simulink subsystem "DirectDriveCycleRefSub"  (R2020b)
settings: Solver=VariableStepAuto  StartTime=0.0  StopTime=10.0  RelTol=1e-3
undefined symbols (not defined in the file): batteryHV, bevMotorSpdRef, motorDrive, vehicle
libraries: autolibshared x1
settings Model: Creator=isaacito  LastModifiedBy=isaacito

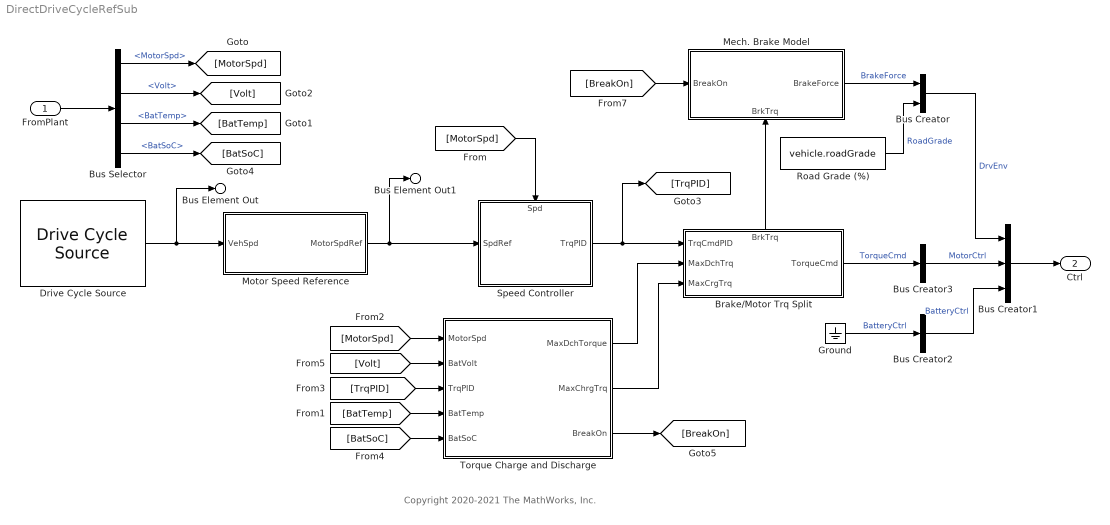
== system DirectDriveCycleRefSub ==
  note: Copyright 2020-2021 The MathWorks, Inc.
  FromPlant : Inport
  Brake/Motor Trq Split : Subsystem
      settings: PortSchema="{\"entries\":[{\"content\":{\"sides\":[{\"content\":{\"connectorIds\":[\"In1\",\"In2\",\"In3\"]},\"type\":\"ConnectorPlacement.EquallySpacedRectSide\",\"uuid\":\"c6883188-188e-4cbf-9dc5-1a26bf01b714\"},{\"content\":{\"connectorIds\":[\"Out1\"],\"side\":\"RIGHT\"},\"type\":\"ConnectorPlacement.EquallySpacedRectSide\",\"uuid\":\"b7c90991-838b-485d-9a4c-3fbacac28b54\"},{\"content\":{\"connectorIds\":[\"Out2\"],\"side\":\"TOP\"},\"type\":\"ConnectorPlacement.EquallySpacedRectSide\",\"uuid\":\"50e43671-3241-4bf5-a3b9-e23b27b7214a\"},{\"content\":{\"connectorIds\":[],\"side\":\"HIDDEN\"},\"type\":\"ConnectorPlacement.EquallySpacedRectSide\",\"uuid\":\"7c25a71e-e9cc-425c-8a3d-1b4aa412427f\"}]},\"type\":\"ConnectorPlacement.EquallySpacedConnector\",\"uuid\":\"d51dcaef-c892-4ef2-982d-c6c52760ceaa\"}],\"packageUris\":[\"http://schema.mathworks.com/mf0/Connector/R2020b\"],\"version\":\"1.0\"}"
  Bus Creator : BusCreator  Inputs=2
  Bus Creator1 : BusCreator  Inputs=3
  Bus Creator2 : BusCreator  Inputs=1
  Bus Creator3 : BusCreator  Inputs=1
  Bus Selector : BusSelector  OutputSignals=Motor.MotorSpd,Battery.Volt,Battery.BatTemp,Battery.BatSoC
  Drive Cycle Source : autolibshared/Drive Cycle Source  cycleVar=FTP75  fileVar=cycleFTP75.mat  tfinal="2474  seconds"  cycleRepeat=off  outAccPort=off  outGearPort=off  gearList=No gear data  t_wot1=5  xdot_woto=0  xdot_wot1=30  t_wot2=20  xdot_wot2=0  t_wotend=30  srcUnit=m/s  outUnit=km/h  srcAccUnit=m/s/s  outAccUnit=m/s^2  dt=0  aMode=1  faultOption=off  velBnd=2  velBndUnit=mph  inUnit=m/s  timeBnd=1  failOption=off  stopSim=off  maxFaultCnt=10  maxFaultTime=2  maxTotFaultTime=15  traceOption=off  dtTrace=1  traceWindow=10  lastDCname=FTP75  lastOutUnit=mph  lastDT=0  lastTB=1  lastSB=2  forceCalcBound=off
      settings: SourceProductBaseCode=PW,MT,VE,VP
  Ground : Ground
  Mech. Brake Model : Subsystem
      settings: PortSchema="{\"entries\":[{\"content\":{\"sides\":[{\"content\":{\"connectorIds\":[\"In1\"]},\"type\":\"ConnectorPlacement.EquallySpacedRectSide\",\"uuid\":\"3fcf8e06-a346-49b8-a4a8-b41cf2b27013\"},{\"content\":{\"connectorIds\":[\"Out1\"],\"side\":\"RIGHT\"},\"type\":\"ConnectorPlacement.EquallySpacedRectSide\",\"uuid\":\"8698242e-d004-4fda-889c-69f0784e7402\"},{\"content\":{\"connectorIds\":[],\"side\":\"TOP\"},\"type\":\"ConnectorPlacement.EquallySpacedRectSide\",\"uuid\":\"7829013b-7288-42bb-bccf-7e6edbe20d12\"},{\"content\":{\"connectorIds\":[\"In2\"],\"side\":\"BOTTOM\"},\"type\":\"ConnectorPlacement.EquallySpacedRectSide\",\"uuid\":\"357a4631-0a09-454f-b0f2-2b693ca62a9f\"},{\"content\":{\"connectorIds\":[],\"side\":\"HIDDEN\"},\"type\":\"ConnectorPlacement.EquallySpacedRectSide\",\"uuid\":\"b5eacf60-b578-4936-bef0-d59a279d5824\"}]},\"type\":\"ConnectorPlacement.EquallySpacedConnector\",\"uuid\":\"d2ebf12e-a3e7-4a55-b8c6-fa4e5ed13b89\"}],\"packageUris\":[\"http://schema.mathworks.com/mf0/Connector/R2020b\"],\"version\":\"1.0\"}"
  Motor Speed Reference : Subsystem
  Road Grade (%) : Constant  Value=vehicle.roadGrade
  Speed Controller : Subsystem
      settings: PortSchema="{\"entries\":[{\"content\":{\"sides\":[{\"content\":{\"connectorIds\":[\"Out1\"]},\"type\":\"ConnectorPlacement.EquallySpacedRectSide\",\"uuid\":\"12b9f2c9-2b28-451b-ad36-7fe4150db485\"},{\"content\":{\"connectorIds\":[\"In2\"],\"side\":\"RIGHT\"},\"type\":\"ConnectorPlacement.EquallySpacedRectSide\",\"uuid\":\"c0fdf9a4-483a-4ddc-b663-6299fcc79327\"},{\"content\":{\"connectorIds\":[\"In1\"],\"side\":\"TOP\"},\"type\":\"ConnectorPlacement.EquallySpacedRectSide\",\"uuid\":\"3f20082e-8487-45e3-9fd7-d6d75741df4d\"}]},\"type\":\"ConnectorPlacement.EquallySpacedConnector\",\"uuid\":\"9361cdd3-74d8-46ee-ae7f-e2dde5d31ed1\"}],\"packageUris\":[\"http://schema.mathworks.com/mf0/Connector/19700101\"],\"version\":\"1.0\"}"
  Torque Charge and Discharge : Subsystem
  Bus Element Out : Outport  PortName=Info  Element=VehSpdRef
      settings: AttributesFormatString=%<Unit>
  Bus Element Out1 : Outport  PortName=Info  Element=MotorSpdRef
      settings: AttributesFormatString=%<Unit>
  Ctrl : Outport  Port=2
  wires:
  Drive Cycle Source/1 -> Bus Element Out/1, Motor Speed Reference/1(VehSpd)
  Motor Speed Reference/1(MotorSpdRef) -> Bus Element Out1/1, Speed Controller/2(SpdRef)
  Road Grade (%)/1 -> Bus Creator/2  "RoadGrade"
  [MotorSpd] -> Speed Controller/1(Spd)
  FromPlant/1 -> Bus Selector/1
  Bus Selector/1 -> [MotorSpd]  "<MotorSpd>"
  Ground/1 -> Bus Creator2/1  "BatteryCtrl"
  Bus Creator/1 -> Bus Creator1/1  "DrvEnv"
  Bus Creator3/1 -> Bus Creator1/2  "MotorCtrl"
  Bus Creator2/1 -> Bus Creator1/3  "BatteryCtrl"
  Bus Creator1/1 -> Ctrl/1
  Bus Selector/2 -> [Volt]  "<Volt>"
  Speed Controller/1(TrqPID) -> Brake/Motor Trq Split/1(TrqCmdPID), [TrqPID]
  Torque Charge and Discharge/3(BreakOn) -> [BreakOn]
  [MotorSpd] -> Torque Charge and Discharge/1(MotorSpd)
  [Volt] -> Torque Charge and Discharge/2(BatVolt)
  [TrqPID] -> Torque Charge and Discharge/3(TrqPID)
  Mech. Brake Model/1(BrakeForce) -> Bus Creator/1  "BrakeForce"
  [BreakOn] -> Mech. Brake Model/1(BreakOn)
  Torque Charge and Discharge/1(MaxDchTorque) -> Brake/Motor Trq Split/2(MaxDchTrq)
  Torque Charge and Discharge/2(MaxChrgTrq) -> Brake/Motor Trq Split/3(MaxCrgTrq)
  Brake/Motor Trq Split/2(BrkTrq) -> Mech. Brake Model/2(BrkTrq)
  Brake/Motor Trq Split/1(TorqueCmd) -> Bus Creator3/1  "TorqueCmd"
  Bus Selector/3 -> [BatTemp]  "<BatTemp>"
  Bus Selector/4 -> [BatSoC]  "<BatSoC>"
  [BatTemp] -> Torque Charge and Discharge/4(BatTemp)
  [BatSoC] -> Torque Charge and Discharge/5(BatSoC)

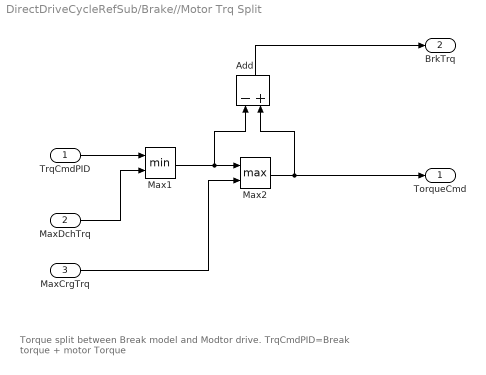
== system DirectDriveCycleRefSub/Brake//Motor Trq Split ==
  note: Torque split between Break model and Modtor drive.
      | TrqCmdPID=Break torque + motor Torque
  TrqCmdPID : Inport
  MaxDchTrq : Inport  Port=2
  MaxCrgTrq : Inport  Port=3
  Add : Sum  Inputs=-+
  Max1 : MinMax  Inputs=2  ZeroCross=off
  Max2 : MinMax  Function=max  Inputs=2  ZeroCross=off
  TorqueCmd : Outport
  BrkTrq : Outport  Port=2
  wires:
  MaxDchTrq/1 -> Max1/2
  Max2/1 -> Add/2, TorqueCmd/1
  Add/1 -> BrkTrq/1
  Max1/1 -> Add/1, Max2/1
  TrqCmdPID/1 -> Max1/1
  MaxCrgTrq/1 -> Max2/2

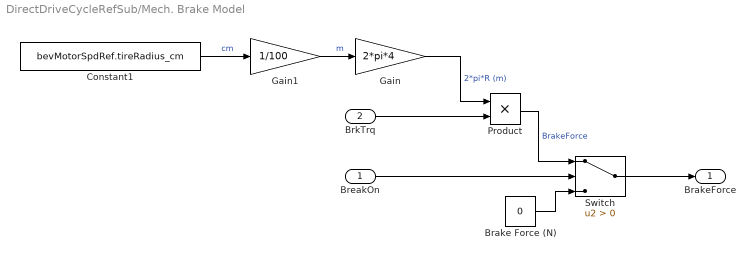
== system DirectDriveCycleRefSub/Mech. Brake Model ==
  BreakOn : Inport
  BrkTrq : Inport  Port=2
  Brake Force (N) : Constant  Value=0
  Constant1 : Constant  Value=bevMotorSpdRef.tireRadius_cm
  Gain : Gain  Gain=2*pi*4
  Gain1 : Gain  Gain=1/100
  Product : Product
  Switch : Switch  Criteria=u2 > Threshold  ZeroCross=off
  BrakeForce : Outport
  wires:
  Switch/1 -> BrakeForce/1
  Gain1/1 -> Gain/1  "m"
  Brake Force (N)/1 -> Switch/3
  BreakOn/1 -> Switch/2
  BrkTrq/1 -> Product/2
  Gain/1 -> Product/1  "2*pi*R (m)"
  Constant1/1 -> Gain1/1  "cm"
  Product/1 -> Switch/1  "BrakeForce"

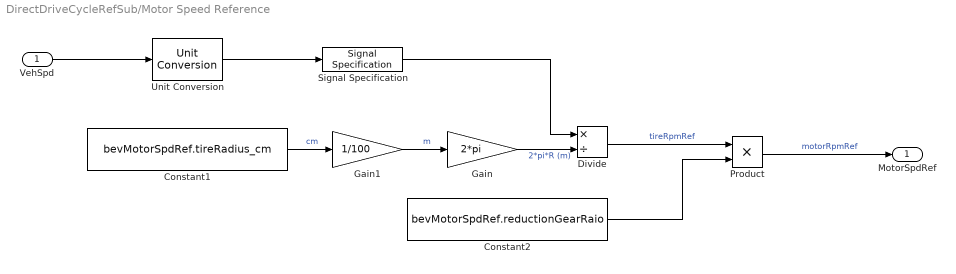
== system DirectDriveCycleRefSub/Motor Speed Reference ==
  VehSpd : Inport  Unit=km/hr
  Constant1 : Constant  Value=bevMotorSpdRef.tireRadius_cm
  Constant2 : Constant  Value=bevMotorSpdRef.reductionGearRaio
  Divide : Product  Inputs=*/
  Gain : Gain  Gain=2*pi
  Gain1 : Gain  Gain=1/100
  Product : Product
  Signal Specification : SignalSpecification  Unit=m/min
  Unit Conversion : UnitConversion
  MotorSpdRef : Outport  Unit=rpm  VectorParamsAs1DForOutWhenUnconnected=off
  wires:
  Gain1/1 -> Gain/1  "m"
  Product/1 -> MotorSpdRef/1  "motorRpmRef"
  Constant2/1 -> Product/2
  Divide/1 -> Product/1  "tireRpmRef"
  Gain/1 -> Divide/2  "2*pi*R (m)"
  Constant1/1 -> Gain1/1  "cm"
  Signal Specification/1 -> Divide/1
  Unit Conversion/1 -> Signal Specification/1
  VehSpd/1 -> Unit Conversion/1

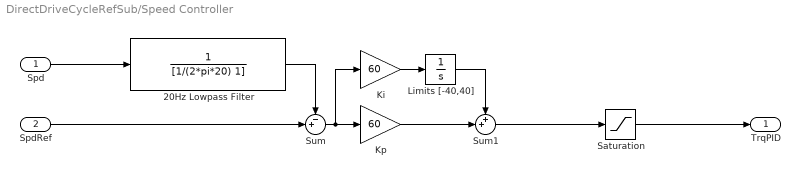
== system DirectDriveCycleRefSub/Speed Controller ==
  Spd : Inport  Unit=rpm
      settings: AttributesFormatString=%<Unit>
  SpdRef : Inport  Port=2  Unit=rpm
      settings: AttributesFormatString=%<Unit>
  20Hz Lowpass Filter : TransferFcn  Denominator=[1/(2*pi*20) 1]
  Ki : Gain  Gain=60
  Kp : Gain  Gain=60
  Limits [-40,40] : Integrator  LimitOutput=on  UpperSaturationLimit=40  LowerSaturationLimit=-40
  Saturation : Saturate  UpperLimit=motorDrive.simplePmsmDrv_trqMax_Nm  LowerLimit=-motorDrive.simplePmsmDrv_trqMax_Nm
      settings: AttributesFormatString=|
      | %<UpperLimit>
      | %<LowerLimit>
  Sum : Sum  Inputs=-+|
  Sum1 : Sum  Inputs=++|
  TrqPID : Outport  Unit=N*m  VectorParamsAs1DForOutWhenUnconnected=off
      settings: AttributesFormatString=%<Unit>
  wires:
  SpdRef/1 -> Sum/2
  Spd/1 -> 20Hz Lowpass Filter/1
  Sum1/1 -> Saturation/1
  Sum/1 -> Ki/1, Kp/1
  Ki/1 -> Limits [-40,40]/1
  Kp/1 -> Sum1/2
  Limits [-40,40]/1 -> Sum1/1
  20Hz Lowpass Filter/1 -> Sum/1
  Saturation/1 -> TrqPID/1

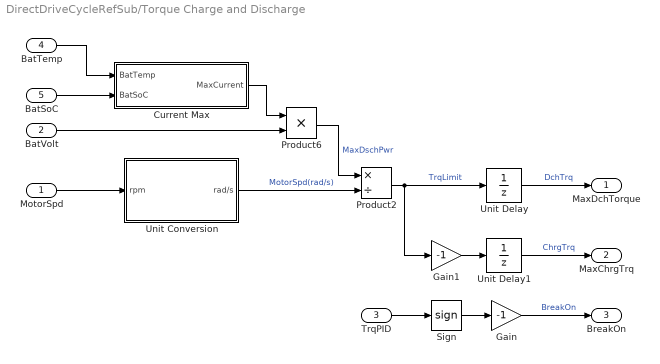
== system DirectDriveCycleRefSub/Torque Charge and Discharge ==
  MotorSpd : Inport
  BatVolt : Inport  Port=2
  TrqPID : Inport  Port=3
  BatTemp : Inport  Port=4
  BatSoC : Inport  Port=5
  Current Max : Subsystem
  Gain : Gain  Gain=-1
  Gain1 : Gain  Gain=-1
  Product2 : Product  Inputs=*/
  Product6 : Product
  Sign : Signum  ZeroCross=off
  Unit Conversion : Subsystem
  Unit Delay : UnitDelay  InitialCondition=eps  SampleTime=-1  HasFrameUpgradeWarning=on
  Unit Delay1 : UnitDelay  InitialCondition=eps  SampleTime=-1  HasFrameUpgradeWarning=on
  MaxDchTorque : Outport
  MaxChrgTrq : Outport  Port=2
  BreakOn : Outport  Port=3
  wires:
  Gain1/1 -> Unit Delay1/1
  Current Max/1(MaxCurrent) -> Product6/1
  BatSoC/1 -> Current Max/2(BatSoC)
  BatTemp/1 -> Current Max/1(BatTemp)
  MotorSpd/1 -> Unit Conversion/1(rpm)
  Unit Conversion/1(rad/s) -> Product2/2  "MotorSpd(rad/s)"
  Product6/1 -> Product2/1  "MaxDschPwr"
  Product2/1 -> Unit Delay/1, Gain1/1  "TrqLimit"
  BatVolt/1 -> Product6/2
  Sign/1 -> Gain/1
  TrqPID/1 -> Sign/1
  Unit Delay1/1 -> MaxChrgTrq/1  "ChrgTrq"
  Gain/1 -> BreakOn/1  "BreakOn"
  Unit Delay/1 -> MaxDchTorque/1  "DchTrq"

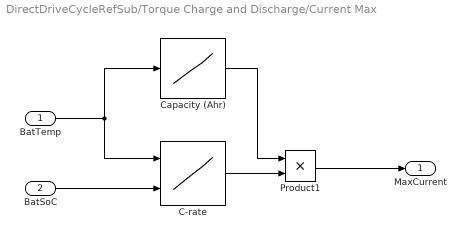
== system DirectDriveCycleRefSub/Torque Charge and Discharge/Current Max ==
  BatTemp : Inport
  BatSoC : Inport  Port=2
  C-rate : Lookup_n-D  BreakpointsForDimension1=batteryHV.batteryTemp_LUT  BreakpointsForDimension2=batteryHV.batterySOC_LUT  Table=batteryHV.cRate'  ExtrapMethod=Clip  UseLastTableValue=on  InternalRulePriority=Speed  RndMeth=Simplest  InputSameDT=on
      settings: InputPortMap=u0,u1
  Capacity (Ahr) : Lookup_n-D  NumberOfTableDimensions=1  BreakpointsForDimension1=batteryHV.batteryTemp_LUT  Table=batteryHV.batteryCapacity_LUT.*batteryHV.batteryNp  ExtrapMethod=Clip  UseLastTableValue=on  InternalRulePriority=Speed  RndMeth=Simplest  InputSameDT=on
  Product1 : Product
  MaxCurrent : Outport
  wires:
  Capacity (Ahr)/1 -> Product1/1
  BatSoC/1 -> C-rate/2
  BatTemp/1 -> Capacity (Ahr)/1, C-rate/1
  Product1/1 -> MaxCurrent/1
  C-rate/1 -> Product1/2

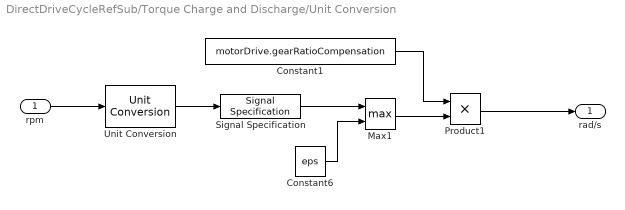
== system DirectDriveCycleRefSub/Torque Charge and Discharge/Unit Conversion ==
  rpm : Inport
  Constant1 : Constant  Value=motorDrive.gearRatioCompensation
  Constant6 : Constant  Value=eps
  Max1 : MinMax  Function=max  Inputs=2  ZeroCross=off
  Product1 : Product
  Signal Specification : SignalSpecification  OutMin=[0]  Unit=rad/sec
  Unit Conversion : UnitConversion
  rad/s : Outport
  wires:
  rpm/1 -> Unit Conversion/1
  Constant1/1 -> Product1/1
  Unit Conversion/1 -> Signal Specification/1
  Max1/1 -> Product1/2
  Product1/1 -> rad/s/1
  Constant6/1 -> Max1/2
  Signal Specification/1 -> Max1/1
